simulink model "PID_StateSpace_CL"  (R2021b)
settings: Solver=VariableStepAuto  StartTime=0.0  StopTime=100  RelTol=1e-3
values from neighbouring files (symbols this model uses):
  C = [0  1  0  0; 0  0  1  0]    [C.mat]
  D = [0 0]    [D.mat]
undefined symbols (not defined in the file or in its folder): Af, Bf, Bwf
libraries: slpidlib x2
settings Model: Creator=stevenfang  LastModifiedBy=stevenfang
settings DebuggingCC: AlgebraicLoopMsg=none

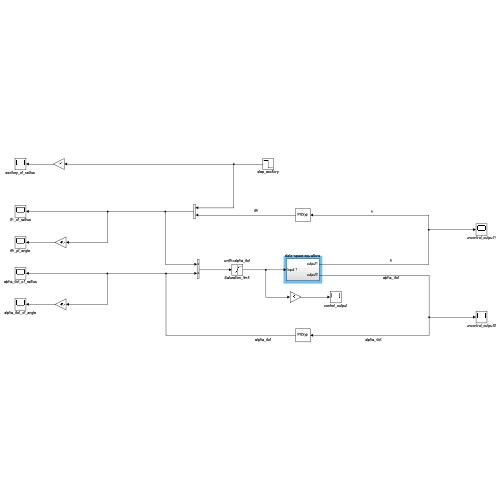
[thumbnail: Simulink's stored preview of the top-level diagram]
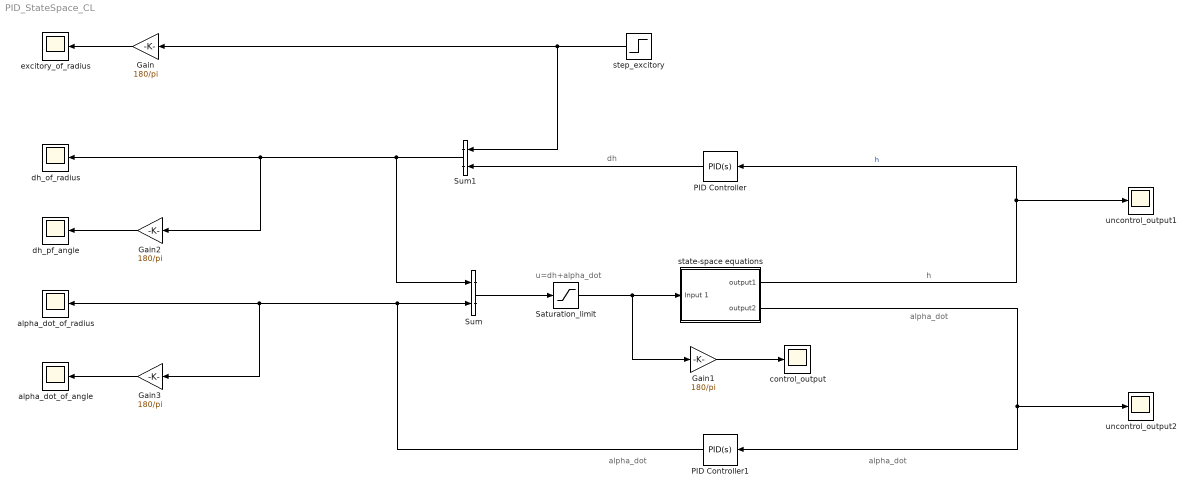
== system PID_StateSpace_CL ==
  note: alpha_dot
  note: h
  note: alpha_dot
  note: dh
  note: u=dh+alpha_dot
  note: alpha_dot
  Gain{,1..3} (4 alike) : Gain  Gain=180/pi
  PID Controller : slpidlib/PID Controller  Controller=PID  Form=Parallel  TimeDomain=Continuous-time  UseExternalTs=off  SampleTime=-1  IntegratorMethod=Forward Euler  FilterMethod=Forward Euler  ControllerParametersSource=internal  P=3.511  I=1.395  D=3.576  UseFilter=on  N=100  TunerSelectOption=Transfer Function Based (PID Tuner App)  InitialConditionSource=internal  InitialConditionForIntegrator=0  InitialConditionForFilter=0  DifferentiatorICPrevScaledInput=0  ExternalReset=none  TrackingMode=off  Kt=1  LimitOutput=off  SatLimitsSource=internal  UpperSaturationLimit=inf  LowerSaturationLimit=-inf  LinearizeAsGain=on  AntiWindupMode=none  Kb=1  POutMin=[]  POutMax=[]  IOutMin=[]  IOutMax=[]  DOutMin=[]  DOutMax=[]  NOutMin=[]  NOutMax=[]  SumOutMin=[]  SumOutMax=[]  SaturationOutMin=[]  SaturationOutMax=[]  PParamMin=[]  PParamMax=[]  IParamMin=[]  IParamMax=[]  DParamMin=[]  DParamMax=[]  NParamMin=[]  NParamMax=[]  KbParamMin=[]  KbParamMax=[]  KtParamMin=[]  KtParamMax=[]  KbOutMin=[]  KbOutMax=[]  KtOutMin=[]  KtOutMax=[]  IntegratorOutMin=[]  IntegratorOutMax=[]  FilterOutMin=[]  FilterOutMax=[]  SumI1OutMin=[]  SumI1OutMax=[]  SumI2OutMin=[]  SumI2OutMax=[]  SumI3OutMin=[]  SumI3OutMax=[]  SumI4OutMin=[]  SumI4OutMax=[]  SumDOutMin=[]  SumDOutMax=[]  DifferentiatorOutMin=[]  DifferentiatorOutMax=[]  FilterDiffOutCoefMin=[]  FilterDiffOutCoefMax=[]  ReciprocalOutMin=[]  ReciprocalOutMax=[]  SumDenOutMin=[]  SumDenOutMax=[]  SumNumOutMin=[]  SumNumOutMax=[]  DivideOutMin=[]  DivideOutMax=[]  UdiffTsProdOutMin=[]  UdiffTsProdOutMax=[]  NTsProdOutMin=[]  NTsProdOutMax=[]  UintegralTsProdOutMin=[]  UintegralTsProdOutMax=[]  UngainTsProdOutMin=[]  UngainTsProdOutMax=[]  IntegratorContinuousStateAttributes=''  IntegratorStateMustResolveToSignalObject=off  IntegratorRTWStateStorageClass=Auto  FilterContinuousStateAttributes=''  FilterStateMustResolveToSignalObject=off  FilterRTWStateStorageClass=Auto  ParallelPVariant=InternalParameters  IdealPVariant=Disabled  IVariant=InternalParameters  DVariant=InternalParameters  IntegratorVariant=Continuous  SatVariant=Disabled  AWVariant=Passthrough  PCopyVariant=Disabled  TRVariant=Disabled  FdbkBlocksVariant=Forward  IdealPFdbkVariant=Disabled  SatFdbkVariant=Disabled  DerivativeFilterVariant=ContFilter  NVariant=InternalParameters  NCopyVariant=Disabled  FilterICVariant=InternalICsFilter  IntegratorICVariant=InternalICs  ExternalResetVariant=Disabled  TRSumVariant=Passthrough  SumFdbkVariant=Disabled  SumVariant=Sum_PID  TsampFilterVariant=InternalTs  TsampNgainVariant=Passthrough  TsampIntegralVariant=Passthrough  ExternalSaturationOutDataTypeStr=Inherit: Same as second input
  PID Controller1 : slpidlib/PID Controller  Controller=PID  Form=Parallel  TimeDomain=Continuous-time  UseExternalTs=off  SampleTime=-1  IntegratorMethod=Forward Euler  FilterMethod=Forward Euler  ControllerParametersSource=internal  P=1.842  I=0  D=0  UseFilter=on  N=100  TunerSelectOption=Transfer Function Based (PID Tuner App)  InitialConditionSource=internal  InitialConditionForIntegrator=0  InitialConditionForFilter=0  DifferentiatorICPrevScaledInput=0  ExternalReset=none  TrackingMode=off  Kt=1  LimitOutput=off  SatLimitsSource=internal  UpperSaturationLimit=inf  LowerSaturationLimit=-inf  LinearizeAsGain=on  AntiWindupMode=none  Kb=1  POutMin=[]  POutMax=[]  IOutMin=[]  IOutMax=[]  DOutMin=[]  DOutMax=[]  NOutMin=[]  NOutMax=[]  SumOutMin=[]  SumOutMax=[]  SaturationOutMin=[]  SaturationOutMax=[]  PParamMin=[]  PParamMax=[]  IParamMin=[]  IParamMax=[]  DParamMin=[]  DParamMax=[]  NParamMin=[]  NParamMax=[]  KbParamMin=[]  KbParamMax=[]  KtParamMin=[]  KtParamMax=[]  KbOutMin=[]  KbOutMax=[]  KtOutMin=[]  KtOutMax=[]  IntegratorOutMin=[]  IntegratorOutMax=[]  FilterOutMin=[]  FilterOutMax=[]  SumI1OutMin=[]  SumI1OutMax=[]  SumI2OutMin=[]  SumI2OutMax=[]  SumI3OutMin=[]  SumI3OutMax=[]  SumI4OutMin=[]  SumI4OutMax=[]  SumDOutMin=[]  SumDOutMax=[]  DifferentiatorOutMin=[]  DifferentiatorOutMax=[]  FilterDiffOutCoefMin=[]  FilterDiffOutCoefMax=[]  ReciprocalOutMin=[]  ReciprocalOutMax=[]  SumDenOutMin=[]  SumDenOutMax=[]  SumNumOutMin=[]  SumNumOutMax=[]  DivideOutMin=[]  DivideOutMax=[]  UdiffTsProdOutMin=[]  UdiffTsProdOutMax=[]  NTsProdOutMin=[]  NTsProdOutMax=[]  UintegralTsProdOutMin=[]  UintegralTsProdOutMax=[]  UngainTsProdOutMin=[]  UngainTsProdOutMax=[]  IntegratorContinuousStateAttributes=''  IntegratorStateMustResolveToSignalObject=off  IntegratorRTWStateStorageClass=Auto  FilterContinuousStateAttributes=''  FilterStateMustResolveToSignalObject=off  FilterRTWStateStorageClass=Auto  ParallelPVariant=InternalParameters  IdealPVariant=Disabled  IVariant=InternalParameters  DVariant=InternalParameters  IntegratorVariant=Continuous  SatVariant=Disabled  AWVariant=Passthrough  PCopyVariant=Disabled  TRVariant=Disabled  FdbkBlocksVariant=Forward  IdealPFdbkVariant=Disabled  SatFdbkVariant=Disabled  DerivativeFilterVariant=ContFilter  NVariant=InternalParameters  NCopyVariant=Disabled  FilterICVariant=InternalICsFilter  IntegratorICVariant=InternalICs  ExternalResetVariant=Disabled  TRSumVariant=Passthrough  SumFdbkVariant=Disabled  SumVariant=Sum_PID  TsampFilterVariant=InternalTs  TsampNgainVariant=Passthrough  TsampIntegralVariant=Passthrough  ExternalSaturationOutDataTypeStr=Inherit: Same as second input
  Saturation_limit : Saturate  UpperLimit=10*(pi/180)  LowerLimit=-10*(pi/180)
  Sum : Sum
  Sum1 : Sum
  alpha_dot_of_angle : Scope
  alpha_dot_of_radius : Scope
  control_output : Scope
  dh_of_radius : Scope
  dh_pf_angle : Scope
  excitory_of_radius : Scope
  state-space equations : Subsystem
  step_excitory : Step  Time=0.1  Before=0.01  After=0  SampleTime=0
  uncontrol_output1 : Scope
  uncontrol_output2 : Scope
  wires:
  state-space equations/1(output1) -> PID Controller/1, uncontrol_output1/1  "h"
  step_excitory/1 -> Gain/1, Sum1/1
  Gain/1 -> excitory_of_radius/1
  Gain1/1 -> control_output/1
  Sum/1 -> Saturation_limit/1
  Saturation_limit/1 -> state-space equations/1(Input 1), Gain1/1
  Sum1/1 -> Gain2/1, dh_of_radius/1, Sum/1
  Gain2/1 -> dh_pf_angle/1
  Gain3/1 -> alpha_dot_of_angle/1
  state-space equations/2(output2) -> PID Controller1/1, uncontrol_output2/1
  PID Controller1/1 -> Sum/2, Gain3/1, alpha_dot_of_radius/1
  PID Controller/1 -> Sum1/2

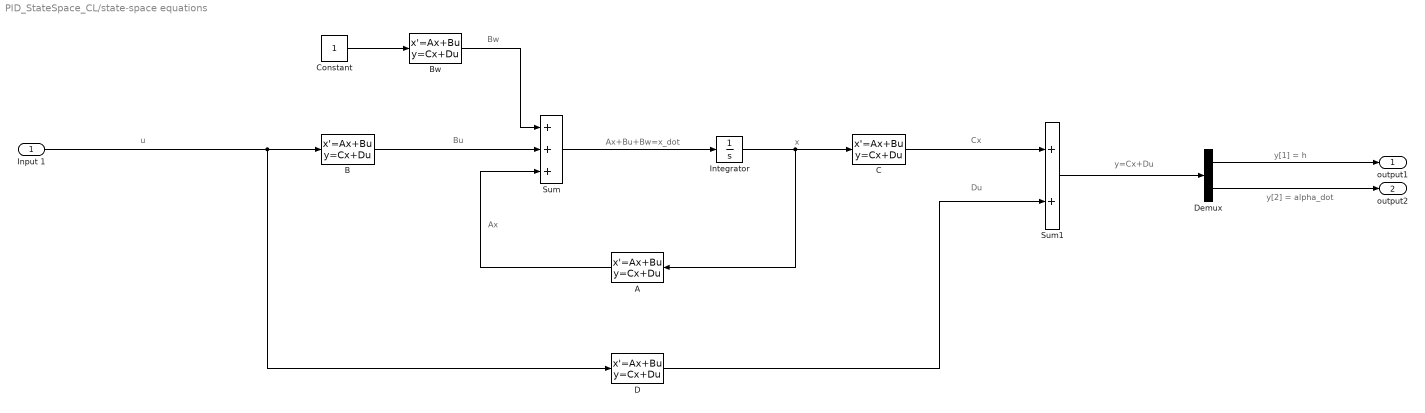
== system PID_StateSpace_CL/state-space equations ==
  note: u
  note: y[2] = alpha_dot
  note: y[1] = h
  note: y=Cx+Du
  note: Du
  note: Cx
  note: Ax
  note: x
  note: Bw
  note: Ax+Bu+Bw=x_dot
  note: Bu
  Input 1 : Inport
  A : StateSpace  A=[]  B=zeros(0,4)  C=zeros(4,0)  D=Af  InitialCondition=0
  B : StateSpace  A=[]  B=zeros(0,1)  C=zeros(4,0)  D=Bf  InitialCondition=0
  Bw : StateSpace  A=[]  B=zeros(0,1)  C=zeros(4,0)  D=Bwf  InitialCondition=0
  C : StateSpace  A=[]  B=zeros(0,4)  C=zeros(2,0)  D=C  InitialCondition=0
  Constant : Constant
  D : StateSpace  A=[]  B=zeros(0,1)  C=zeros(2,0)  D=D  InitialCondition=0
  Demux : Demux  Outputs=2
  Integrator : Integrator
  Sum : Sum  Inputs=+++
  Sum1 : Sum
  output1 : Outport
  output2 : Outport  Port=2
  wires:
  Demux/1 -> output1/1
  A/1 -> Sum/3
  C/1 -> Sum1/1
  B/1 -> Sum/2
  Demux/2 -> output2/1
  Bw/1 -> Sum/1
  D/1 -> Sum1/2
  Sum/1 -> Integrator/1
  Input 1/1 -> D/1, B/1
  Sum1/1 -> Demux/1
  Integrator/1 -> A/1, C/1
  Constant/1 -> Bw/1
